simulink model "Teleoperation_Task_Space"  (R2021b)
settings: Solver=FixedStepAuto  StartTime=0.0  StopTime=20  FixedStep=Ts  RelTol=1e-3
values from neighbouring files (symbols this model uses):
  alphas_m = 75.0 * ones(1,dh.dof_task)    [setup_teleop.m]
  alphas_s = alphas_m    [setup_teleop.m]
  B_m = diag(ones(1,dh.dof_task)) * 100    [setup_teleop.m]
  B_s = diag(ones(1,dh.dof_task)) * 15    [setup_teleop.m]
  Fh_A = [1 4*wc 6*wc^2 4*wc^3 wc^4]    [setup_teleop.m]
  Fh_B = [0 0 0 0 wc^4]    [setup_teleop.m]
  gravity = [0 0 9.81]'    [setup_robot.m]
  K_g = eye(dh.dof_task) * k_g    [setup_teleop.m]
  K_m = diag(ones(1,dh.dof_task)) * 0    [setup_teleop.m]
  K_s = diag(ones(1,dh.dof_task)) * 75    [setup_teleop.m]
  KD_e = zeros(dh.dof_task); KD_e(1,1) = 10    [setup_teleop.m]
  KD_h = eye(dh.dof_task) * 50.0    [setup_teleop.m]
  KE_e = zeros(dh.dof_task); KE_e(1,1) = 100    [setup_teleop.m]
  KP_h = eye(dh.dof_task) * 350.0    [setup_teleop.m]
  lambdas_m = 4.0 * ones(1,dh.dof_task)    [setup_teleop.m]
  lambdas_s = lambdas_m    [setup_teleop.m]
  M_m = diag(ones(1,dh.dof_task)) * 1    [setup_teleop.m]
  M_s = diag(ones(1,dh.dof_task)) * 1    [setup_teleop.m]
  T_m2s = 25 / 1000 / Ts    (= 25)    [setup_teleop.m]
  T_s2m = 25 / 1000 / Ts    (= 25)    [setup_teleop.m]
  td = [            0            1                          10            18 ]    [setup_teleop.m]
  Xe = conf.init.x0    [setup_teleop.m]
  zdq_A = [1 4*wc 6*wc^2 4*wc^3 wc^4]    [setup_teleop.m]
  zdq_B = [0 0 0 0 wc^4]    [setup_teleop.m]
undefined symbols (not defined in the file or in its folder): conf_m, conf_s, dh, Fm_A, Fm_B, Fs_A, Fs_B, x0
libraries: vrlib x2, robotcorelib x1, simulink x1
(part 1 of 2)
settings Model: Creator=eros  LastModifiedBy=Sebastiano
settings SolverCC: AlgebraicLoopSolver=TrustRegion
settings DebuggingCC: SFMachineParentedDataDiag=warning

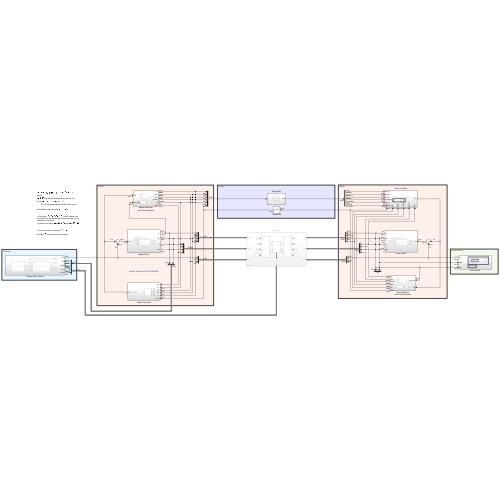
[thumbnail: Simulink's stored preview of the top-level diagram]
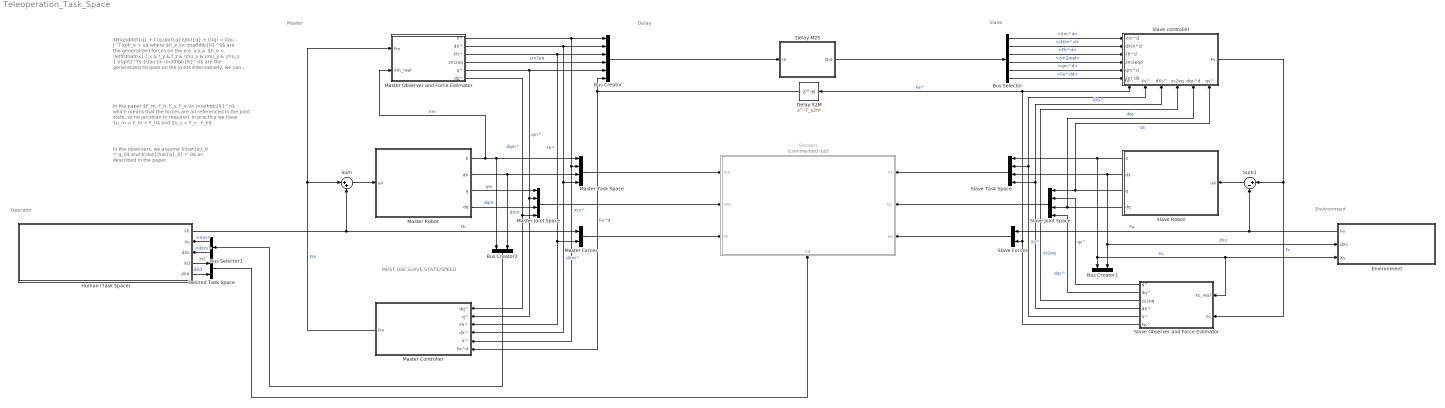
== system Teleoperation_Task_Space ==
  note: MUST USE SLAVE STATE/SPEED
  note: Operator
  note: Environment
  note: Delay
  note: Master
  note: Slave
  note: In the observers, we assume $\hat{q}_0 = q_0$ and $\dot{\hat{q}_0} = 0$ as described in the paper.
  note: In the paper $F_m, F_h, F_s, F_e \in \mathbb{R}^n$ , which means that the forces are all referenced in the joint state, so no Jacobian in required.
      | In practice we have $u_m = F_m + F_h$ and $u_s = F_s - F_e$
  note: $B(q)\ddot{q} + C(q,\dot{q})\dot{q} + G(q) = \tau - J^T(q)h_e = u$
      | where
      | $h_e \in \mathbb{R}^6$ are the generalized forces on the e.e.
      | a.k.a. $h_e = \left[\matrix{ f_x & f_y & f_z & \mu_x & \mu_y & \mu_z } \right]^T$
      | $\tau \in \mathbb{R}^n$ are the generalized torques on the joints
      |
      | Alternatively, we can write $\tau = J^T(q)\tau_e$ .
  Bus Creator : BusCreator  Inputs=6
  Bus Creator1 : BusCreator  Inputs=2
  Bus Creator2 : BusCreator  Inputs=2
  Bus Selector : BusSelector  OutputSignals=Xm^d,dXm^d,Fh^d,zm2eqd,qm^d,Fe^dd
  Bus Selector1 : BusSelector  OutputSignals=Xm,dXm
  Delay M2S : Subsystem
  Delay S2M : Delay  DelayLength=T_s2m
  Desired Task Space : BusCreator  Inputs=2
  Environment : Subsystem
      settings: PortSchema="{\"entries\":[{\"content\":{\"sides\":[{\"content\":{\"connectorIds\":[\"Out1\",\"In1\",\"In2\"]},\"type\":\"ConnectorPlacement.EquallySpacedRectSide\",\"uuid\":\"3a683f5f-8229-405f-b97f-b506986b9524\"},{\"content\":{\"connectorIds\":[],\"side\":\"RIGHT\"},\"type\":\"ConnectorPlacement.EquallySpacedRectSide\",\"uuid\":\"ee737040-7d2a-42b5-b72e-c46d7dc1a0a9\"},{\"content\":{\"connectorIds\":[],\"side\":\"TOP\"},\"type\":\"ConnectorPlacement.EquallySpacedRectSide\",\"uuid\":\"297da6e9-ed01-499d-b3c2-0f0e3cad7b3e\"}]},\"type\":\"ConnectorPlacement.EquallySpacedConnector\",\"uuid\":\"c177a36f-944e-4ac9-b62c-2e9de2d24660\"}],\"packageUris\":[\"http://schema.mathworks.com/mf0/Connector/R2020b\"],\"version\":\"1.0\"}"
  Human (Task Space) : Subsystem
      settings: PortSchema="{\"entries\":[{\"content\":{\"sides\":[{\"content\":{\"connectorIds\":[]},\"type\":\"ConnectorPlacement.EquallySpacedRectSide\",\"uuid\":\"7778f5b7-85d4-4afc-857c-056ec77f7c35\"},{\"content\":{\"connectorIds\":[\"Out1\",\"In1\",\"In2\",\"Out2\",\"Out3\"],\"side\":\"RIGHT\"},\"type\":\"ConnectorPlacement.EquallySpacedRectSide\",\"uuid\":\"4e6a4d83-f8e8-4554-84b1-926a6f2c9c17\"},{\"content\":{\"connectorIds\":[],\"side\":\"TOP\"},\"type\":\"ConnectorPlacement.EquallySpacedRectSide\",\"uuid\":\"7c53f63a-15b9-4620-895a-15c4690edfa5\"}]},\"type\":\"ConnectorPlacement.EquallySpacedConnector\",\"uuid\":\"f47fbd83-fa7b-4372-bf8b-e8c7b2e83c33\"}],\"packageUris\":[\"http://schema.mathworks.com/mf0/Connector/R2020b\"],\"version\":\"1.0\"}"
  Master Controller : Subsystem
  Master Forces : BusCreator  Inputs=2
  Master Joint Space : BusCreator  Inputs=4
  Master Observer and Force Estimator : Subsystem
  Master Robot : Subsystem
  Master Task Space : BusCreator  Inputs=4
  Sensors : Subsystem  Commented=on
      settings: PortSchema="{\"entries\":[{\"content\":{\"sides\":[{\"content\":{\"connectorIds\":[\"In1\",\"In2\",\"In3\"]},\"type\":\"ConnectorPlacement.EquallySpacedRectSide\",\"uuid\":\"54c087a6-e628-45a0-8beb-ec377517c1fd\"},{\"content\":{\"connectorIds\":[\"In5\",\"In6\",\"In7\"],\"side\":\"RIGHT\"},\"type\":\"ConnectorPlacement.EquallySpacedRectSide\",\"uuid\":\"42defee6-bb8f-41f0-bcac-2060d15fab8b\"},{\"content\":{\"connectorIds\":[],\"side\":\"TOP\"},\"type\":\"ConnectorPlacement.EquallySpacedRectSide\",\"uuid\":\"25403ab0-b6a1-4ec4-8138-b166c3bde76b\"},{\"content\":{\"connectorIds\":[\"In4\"],\"side\":\"BOTTOM\"},\"type\":\"ConnectorPlacement.EquallySpacedRectSide\",\"uuid\":\"d9d00fac-eb94-4801-95c9-2f27ca054ba8\"}]},\"type\":\"ConnectorPlacement.EquallySpacedConnector\",\"uuid\":\"2fd4c0cb-09a7-477d-a6ac-6df7d0139477\"}],\"packageUris\":[\"http://schema.mathworks.com/mf0/Connector/R2020b\"],\"version\":\"1.0\"}"
  Slave Forces : BusCreator  Inputs=2
  Slave Joint Space : BusCreator  Inputs=4
  Slave Observer and Force Estimator : Subsystem
  Slave Robot : Subsystem
  Slave Task Space : BusCreator  Inputs=4
  Slave controller : Subsystem
      settings: PortSchema="{\"entries\":[{\"content\":{\"sides\":[{\"content\":{\"connectorIds\":[\"In1\",\"In2\",\"In3\",\"In4\",\"In5\",\"In6\"]},\"type\":\"ConnectorPlacement.EquallySpacedRectSide\",\"uuid\":\"b1f66af2-ed99-40b6-8cf8-b97c23f93a67\"},{\"content\":{\"connectorIds\":[\"Out1\"],\"side\":\"RIGHT\"},\"type\":\"ConnectorPlacement.EquallySpacedRectSide\",\"uuid\":\"bd8dc41a-d4bd-4421-a4e6-8b9f2d2ea86c\"},{\"content\":{\"connectorIds\":[],\"side\":\"TOP\"},\"type\":\"ConnectorPlacement.EquallySpacedRectSide\",\"uuid\":\"bc806d3a-77b0-4d29-b087-7d48d5aabf51\"},{\"content\":{\"connectorIds\":[\"In7\",\"In8\",\"In9\",\"In10\",\"In11\",\"In12\"],\"side\":\"BOTTOM\"},\"type\":\"ConnectorPlacement.EquallySpacedRectSide\",\"uuid\":\"ca1d5307-1d0f-4028-b8dc-88a57f95ff6b\"}]},\"type\":\"ConnectorPlacement.EquallySpacedConnector\",\"uuid\":\"a48c829b-f218-4f75-a112-dfe3646c5e86\"}],\"packageUris\":[\"http://schema.mathworks.com/mf0/Connector/R2020b\"],\"version\":\"1.0\"}"
  Sum : Sum  Inputs=|++
  Sum1 : Sum  Inputs=|+-
  wires:
  Slave Observer and Force Estimator/1(q^) -> Slave Joint Space/2  "qs^"
  Slave Observer and Force Estimator/3(zs2eq) -> Slave controller/10(zs2eq)  "zs2eq"
  Master Observer and Force Estimator/1(X^) -> Master Task Space/2, Master Controller/5(X^), Bus Creator/1  "Xm^"
  Slave Observer and Force Estimator/6(Fe^) -> Delay S2M/1, Slave controller/7(Fe^), Slave Forces/2  "Fe^"
  Master Observer and Force Estimator/3(Fh^) -> Bus Creator/3, Master Controller/3(Fh^), Master Forces/2  "Fh^"
  Slave Observer and Force Estimator/2(dq^) -> Slave Joint Space/4  "dqs^"
  Master Observer and Force Estimator/2(dX^) -> Bus Creator/2, Master Task Space/4, Master Controller/4(dX^)  "dXm^"
  Master Controller/1(Fm) -> Master Observer and Force Estimator/1(Fm), Sum/1  "Fm"
  Slave controller/1(Fs) -> Slave Observer and Force Estimator/2(Fs), Sum1/1  "Fs"
  Master Observer and Force Estimator/4(zm2eq) -> Bus Creator/4  "zm2eq"
  Bus Selector/6 -> Slave controller/6(Fe^dd)  "<Fe^dd>"
  Bus Selector/2 -> Slave controller/2(dXm^d)  "<dXm^d>"
  Bus Selector/1 -> Slave controller/1(Xm^d)  "<Xm^d>"
  Bus Selector/3 -> Slave controller/3(Fh^d)  "<Fh^d>"
  Bus Selector/4 -> Slave controller/4(zm2eqd)  "<zm2eqd>"
  Delay S2M/1 -> Bus Creator/6, Master Controller/6(Fe^d)  "Fe^d"
  Slave Robot/3(q) -> Slave Joint Space/1, Slave controller/12(qs^)  "qs"
  Slave Robot/4(dq) -> Slave Joint Space/3, Slave controller/11(dqs^d)  "dqs"
  Master Robot/1(X) -> Bus Creator2/1, Master Task Space/1, Master Observer and Force Estimator/2(Xm_real)  "Xm"
  Human (Task Space)/1(Fh) -> Sum/2, Master Forces/1  "Fh"
  Sum/1 -> Master Robot/1(uA)
  Master Robot/3(q) -> Master Joint Space/1  "qm"
  Master Observer and Force Estimator/5(q^) -> Bus Creator/5, Master Controller/2(q^), Master Joint Space/2  "qm^"
  Master Observer and Force Estimator/6(dq^) -> Master Controller/1(dq^), Master Joint Space/4  "dqm^"
  Master Robot/4(dq) -> Master Joint Space/3  "dqm"
  Master Robot/2(dX) -> Master Task Space/3, Bus Creator2/2  "dXm"
  Sum1/1 -> Slave Robot/1(uA)
  Slave Robot/1(X) -> Slave Observer and Force Estimator/1(Xs_real), Environment/2(Xs), Bus Creator1/1, Slave Task Space/1  "Xs"
  Slave Robot/2(dX) -> Slave Task Space/3, Environment/1(dXs), Bus Creator1/2  "dXs"
  Slave Observer and Force Estimator/5(X^) -> Slave controller/8(Xs^), Slave Task Space/2  "Xs^"
  Slave Observer and Force Estimator/4(dX^) -> Slave Task Space/4, Slave controller/9(dXs^)  "dXs^"
  Bus Selector/5 -> Slave controller/5(qm^d)  "<qm^d>"
  Environment/1(Fe) -> Sum1/2, Slave Forces/1  "Fe"
  Human (Task Space)/2(Xd) -> Desired Task Space/1  "Xd"
  Human (Task Space)/3(dXd) -> Desired Task Space/2  "dXd"
  Master Task Space/1 -> Sensors/1(Xm)
  Slave Task Space/1 -> Sensors/5(Xs)
  Master Joint Space/1 -> Sensors/2(Qm)
  Slave Joint Space/1 -> Sensors/6(Qs)
  Master Forces/1 -> Sensors/3(Fh)
  Slave Forces/1 -> Sensors/7(Fe)
  Desired Task Space/1 -> Sensors/4(Xd)
  Bus Selector1/2 -> Human (Task Space)/2(dXs)  "<dXm>"
  Bus Selector1/1 -> Human (Task Space)/1(Xs)  "<Xm>"
  Bus Creator2/1 -> Bus Selector1/1
  Bus Creator/1 -> Delay M2S/1(In)
  Delay M2S/1(Out) -> Bus Selector/1

== system Teleoperation_Task_Space/Delay M2S ==
  note: Initial conditions of the delays are set to be the initial condition of the slave robot.
      | When the first signal from the master is received, the slave follows it immediately.
  In : Inport
  Bus Creator3 : BusCreator  Inputs=6
  Bus Selector2 : BusSelector  OutputSignals=Xm^,dXm^,Fh^,zm2eq,qm^,Fe^d
  Delay M2S : Delay  DelayLength=T_m2s  InitialCondition=repmat(conf_s.init.x0, [1,1,T_m2s])
  Delay M2S1 : Delay  DelayLength=T_m2s
  Delay M2S2 : Delay  DelayLength=T_m2s  InitialCondition=repmat(conf_s.init.q0, [1,T_m2s])
  Delay M2S3 : Delay  DelayLength=T_m2s
  Delay M2S4 : Delay  DelayLength=T_m2s
  Delay M2S5 : Delay  DelayLength=T_m2s  InitialCondition=repmat(conf_s.init.dx0, [1,1,T_m2s])
  Out : Outport
  wires:
  Delay M2S4/1 -> Bus Creator3/3  "Fh^d"
  Bus Selector2/4 -> Delay M2S3/1  "<zm2eq>"
  Delay M2S2/1 -> Bus Creator3/5  "qm^d"
  Delay M2S3/1 -> Bus Creator3/4  "zm2eqd"
  Bus Selector2/1 -> Delay M2S/1  "<Xm^>"
  Bus Selector2/5 -> Delay M2S2/1  "<qm^>"
  Delay M2S5/1 -> Bus Creator3/2  "dXm^d"
  Bus Selector2/6 -> Delay M2S1/1  "<Fe^d>"
  Delay M2S1/1 -> Bus Creator3/6  "Fe^dd"
  Bus Selector2/2 -> Delay M2S5/1  "<dXm^>"
  Bus Selector2/3 -> Delay M2S4/1  "<Fh^>"
  Delay M2S/1 -> Bus Creator3/1  "Xm^d"
  In/1 -> Bus Selector2/1
  Bus Creator3/1 -> Out/1

== system Teleoperation_Task_Space/Environment ==
  note: No Environment
  note: Spring Environment
  note: Spring-Damper Environment
  dXs : Inport
  Xs : Inport  Port=2
  Constant1 : Constant  Value=zeros(1,dh.dof_task)
  Constant2 : Constant  Value=zeros(1,dh.dof_task)
  Constant4 : Constant  Value=Xe
  Manual Switch : ManualSwitch
  Manual Switch1 : ManualSwitch
  Multiply : Gain  Gain=KE_e  Multiplication=Matrix(K*u)
  Multiply1 : Gain  Gain=KD_e  Multiplication=Matrix(K*u)
  Product : Product
  Subsystem : Subsystem
  Sum : Sum  Inputs=|++
  Fe : Outport
  wires:
  Product/1 -> Manual Switch/1
  Constant1/1 -> Manual Switch1/2
  Manual Switch/1 -> Fe/1
  Multiply/1 -> Sum/1
  Manual Switch1/1 -> Sum/2
  Multiply1/1 -> Manual Switch1/1
  dXs/1 -> Multiply1/1
  Constant2/1 -> Manual Switch/2
  Constant4/1 -> Subsystem/2(EnvironmentPose)
  Xs/1 -> Subsystem/1(SlavePose)
  Subsystem/1(IsTouching) -> Product/1
  Sum/1 -> Product/2
  Subsystem/2(Displacement) -> Multiply/1

== system Teleoperation_Task_Space/Human (Task Space) ==
  Xs : Inport
  dXs : Inport  Port=2
  Motion Tracking control : Subsystem
      settings: PortSchema="{\"entries\":[{\"content\":{\"sides\":[{\"content\":{\"connectorIds\":[\"In1\",\"In2\",\"In3\"]},\"type\":\"ConnectorPlacement.EquallySpacedRectSide\",\"uuid\":\"52575601-e286-4809-a30d-cedf982d9693\"},{\"content\":{\"connectorIds\":[\"Out1\",\"In4\",\"In5\"],\"side\":\"RIGHT\"},\"type\":\"ConnectorPlacement.EquallySpacedRectSide\",\"uuid\":\"ad2168cb-d0b7-4f4a-9914-0c84d01558f7\"},{\"content\":{\"connectorIds\":[],\"side\":\"TOP\"},\"type\":\"ConnectorPlacement.EquallySpacedRectSide\",\"uuid\":\"311024f8-e557-4a51-82a2-8dec63492c2b\"}]},\"type\":\"ConnectorPlacement.EquallySpacedConnector\",\"uuid\":\"f15c02cd-b134-4f17-b903-786a9234fd9d\"}],\"packageUris\":[\"http://schema.mathworks.com/mf0/Connector/R2020b\"],\"version\":\"1.0\"}"
  Task Space trajectory : Subsystem
  Fh : Outport
  Xd : Outport  Port=2
  dXd : Outport  Port=3
  wires:
  Task Space trajectory/2(dXd) -> dXd/1, Motion Tracking control/2(dXd)
  dXs/1 -> Motion Tracking control/4(dXs)
  Motion Tracking control/1(uA) -> Fh/1
  Xs/1 -> Motion Tracking control/5(Xs)
  Task Space trajectory/3(Xd) -> Xd/1, Motion Tracking control/3(Xd)
  Task Space trajectory/1(ddXd) -> Motion Tracking control/1(ddXd)

== system Teleoperation_Task_Space/Master Controller ==
  note: Here we provide q^ and dq^ just to avoid calculating them
  dq^ : Inport
  q^ : Inport  Port=2
  Fh^ : Inport  Port=3
  dX^ : Inport  Port=4
  X^ : Inport  Port=5
  Fe^d : Inport  Port=6
  Master Command Filter : Subsystem  Commented=through  TreatAsAtomicUnit=on
  Master Controller : MATLAB Function  TreatAsAtomicUnit=on
  Fm : Outport
  wires:
  Fh^/1 -> Master Controller/5(Fh)
  Fe^d/1 -> Master Controller/6(Fe_d)
  Master Controller/1(Fm) -> Master Command Filter/1(In1)
  X^/1 -> Master Controller/3(Xm)
  dX^/1 -> Master Controller/4(dXm)
  dq^/1 -> Master Controller/2(dqm)
  q^/1 -> Master Controller/1(qm)
  Master Command Filter/1(Out1) -> Fm/1

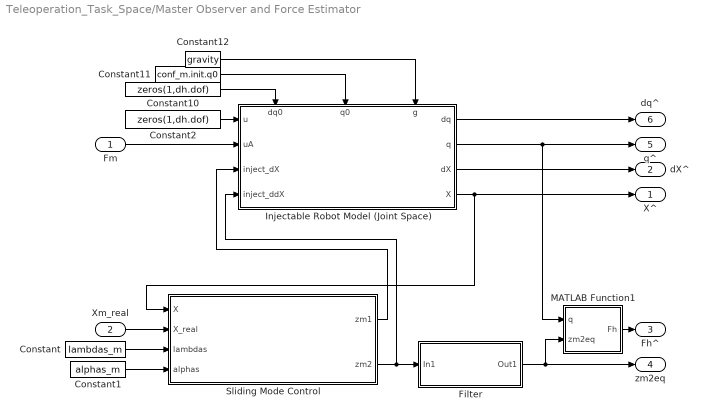
== system Teleoperation_Task_Space/Master Observer and Force Estimator ==
  Fm : Inport
  Xm_real : Inport  Port=2
  Constant : Constant  Value=lambdas_m
  Constant1 : Constant  Value=alphas_m
  Constant10 : Constant  Value=zeros(1,dh.dof)
  Constant11 : Constant  Value=conf_m.init.q0
  Constant12 : Constant  Value=gravity
  Constant2 : Constant  Value=zeros(1,dh.dof)
  Filter : Subsystem  TreatAsAtomicUnit=on
  Injectable Robot Model (Joint Space) : Subsystem
      settings: PortSchema="{\"entries\":[{\"content\":{\"sides\":[{\"content\":{\"connectorIds\":[\"In1\",\"In2\",\"In3\",\"In4\"]},\"type\":\"ConnectorPlacement.EquallySpacedRectSide\",\"uuid\":\"a8701c64-329e-4144-b882-ecf5d621aff2\"},{\"content\":{\"connectorIds\":[\"Out1\",\"Out2\",\"Out3\",\"Out4\"],\"side\":\"RIGHT\"},\"type\":\"ConnectorPlacement.EquallySpacedRectSide\",\"uuid\":\"4e168703-1cb9-438c-bc6b-9b2d7fbb809e\"},{\"content\":{\"connectorIds\":[\"In5\",\"In6\",\"In7\"],\"side\":\"TOP\"},\"type\":\"ConnectorPlacement.EquallySpacedRectSide\",\"uuid\":\"8fbcb29e-7fab-4224-b4ad-ee01c13d675a\"}]},\"type\":\"ConnectorPlacement.EquallySpacedConnector\",\"uuid\":\"fa721fab-1ce6-4fdf-95fa-8ada3ed2d65c\"}],\"packageUris\":[\"http://schema.mathworks.com/mf0/Connector/R2020b\"],\"version\":\"1.0\"}"
  MATLAB Function1 : MATLAB Function  TreatAsAtomicUnit=on
  Sliding Mode Control : Subsystem
  X^ : Outport
  dX^ : Outport  Port=2
  Fh^ : Outport  Port=3
  zm2eq : Outport  Port=4
  q^ : Outport  Port=5
  dq^ : Outport  Port=6
  wires:
  Filter/1(Out1) -> MATLAB Function1/2(zm2eq), zm2eq/1
  Sliding Mode Control/1(zm1) -> Injectable Robot Model (Joint Space)/3(inject_dX)
  Sliding Mode Control/2(zm2) -> Filter/1(In1), Injectable Robot Model (Joint Space)/4(inject_ddX)
  Constant1/1 -> Sliding Mode Control/4(alphas)
  Constant/1 -> Sliding Mode Control/3(lambdas)
  Xm_real/1 -> Sliding Mode Control/2(X_real)
  Injectable Robot Model (Joint Space)/4(X) -> X^/1, Sliding Mode Control/1(X)
  Injectable Robot Model (Joint Space)/3(dX) -> dX^/1
  Constant11/1 -> Injectable Robot Model (Joint Space)/6(q0)
  Constant10/1 -> Injectable Robot Model (Joint Space)/5(dq0)
  Injectable Robot Model (Joint Space)/1(dq) -> dq^/1
  Constant12/1 -> Injectable Robot Model (Joint Space)/7(g)
  Injectable Robot Model (Joint Space)/2(q) -> MATLAB Function1/1(q), q^/1
  MATLAB Function1/1(Fh) -> Fh^/1
  Constant2/1 -> Injectable Robot Model (Joint Space)/1(u)
  Fm/1 -> Injectable Robot Model (Joint Space)/2(uA)

== system Teleoperation_Task_Space/Master Robot ==
  uA : Inport
  Constant1 : Constant  Value=zeros(1,dh.dof)
  Constant10 : Constant  Value=conf_m.init.dq0
  Constant11 : Constant  Value=conf_m.init.q0
  Constant12 : Constant  Value=gravity
  Constant2 : Constant  Value=zeros(1,dh.dof_task)
  Injectable Robot Model (Joint Space) : Subsystem
      settings: PortSchema="{\"entries\":[{\"content\":{\"sides\":[{\"content\":{\"connectorIds\":[\"In1\",\"In2\",\"In3\",\"In4\"]},\"type\":\"ConnectorPlacement.EquallySpacedRectSide\",\"uuid\":\"a8701c64-329e-4144-b882-ecf5d621aff2\"},{\"content\":{\"connectorIds\":[\"Out1\",\"Out2\",\"Out3\",\"Out4\"],\"side\":\"RIGHT\"},\"type\":\"ConnectorPlacement.EquallySpacedRectSide\",\"uuid\":\"4e168703-1cb9-438c-bc6b-9b2d7fbb809e\"},{\"content\":{\"connectorIds\":[\"In5\",\"In6\",\"In7\"],\"side\":\"TOP\"},\"type\":\"ConnectorPlacement.EquallySpacedRectSide\",\"uuid\":\"8fbcb29e-7fab-4224-b4ad-ee01c13d675a\"}]},\"type\":\"ConnectorPlacement.EquallySpacedConnector\",\"uuid\":\"fa721fab-1ce6-4fdf-95fa-8ada3ed2d65c\"}],\"packageUris\":[\"http://schema.mathworks.com/mf0/Connector/R2020b\"],\"version\":\"1.0\"}"
  X : Outport
  dX : Outport  Port=2
  q : Outport  Port=3
  dq : Outport  Port=4
  wires:
  Constant10/1 -> Injectable Robot Model (Joint Space)/5(dq0)
  Constant2/1 -> Injectable Robot Model (Joint Space)/4(inject_ddX), Injectable Robot Model (Joint Space)/3(inject_dX)
  Constant11/1 -> Injectable Robot Model (Joint Space)/6(q0)
  Injectable Robot Model (Joint Space)/2(q) -> q/1
  Injectable Robot Model (Joint Space)/3(dX) -> dX/1
  Constant12/1 -> Injectable Robot Model (Joint Space)/7(g)
  Injectable Robot Model (Joint Space)/4(X) -> X/1
  Injectable Robot Model (Joint Space)/1(dq) -> dq/1
  uA/1 -> Injectable Robot Model (Joint Space)/2(uA)
  Constant1/1 -> Injectable Robot Model (Joint Space)/1(u)

== system Teleoperation_Task_Space/Sensors ==
  Xm : Inport
  Qm : Inport  Port=2
  Fh : Inport  Port=3
  Xd : Inport  Port=4
  Xs : Inport  Port=5
  Qs : Inport  Port=6
  Fe : Inport  Port=7
  Compare Sensors : Subsystem
      settings: PortSchema="{\"entries\":[{\"content\":{\"sides\":[{\"content\":{\"connectorIds\":[\"In1\",\"In2\"]},\"type\":\"ConnectorPlacement.EquallySpacedRectSide\",\"uuid\":\"eee4eb85-6cb8-4462-85fc-1aafb3c3937f\"},{\"content\":{\"connectorIds\":[\"In4\",\"In5\"],\"side\":\"RIGHT\"},\"type\":\"ConnectorPlacement.EquallySpacedRectSide\",\"uuid\":\"5ab37ec6-6ee1-47e9-aff6-41baaee9b59b\"},{\"content\":{\"connectorIds\":[],\"side\":\"TOP\"},\"type\":\"ConnectorPlacement.EquallySpacedRectSide\",\"uuid\":\"6f11ee79-2d90-4b50-8360-b99d360f33b3\"},{\"content\":{\"connectorIds\":[\"In3\"],\"side\":\"BOTTOM\"},\"type\":\"ConnectorPlacement.EquallySpacedRectSide\",\"uuid\":\"fafd6e14-ac6f-4eee-8610-fc1b1c686699\"}]},\"type\":\"ConnectorPlacement.EquallySpacedConnector\",\"uuid\":\"5676dc65-12f4-4a54-a0ce-a07c6c462ad2\"}],\"packageUris\":[\"http://schema.mathworks.com/mf0/Connector/R2020b\"],\"version\":\"1.0\"}"
  Master Desired Pose : Subsystem
  Master Sensors : Subsystem
  Slave Desired Pose : Subsystem
  Slave Sensors : Subsystem
  wires:
  Xd/1 -> Compare Sensors/3(Xd)
  Slave Sensors/2(dXs) -> Compare Sensors/5(dXs)
  Master Sensors/2(dXm) -> Compare Sensors/2(dXm)
  Fh/1 -> Master Sensors/3(F)
  Fe/1 -> Slave Sensors/3(F)
  Qs/1 -> Slave Sensors/2(Q)
  Xm/1 -> Master Sensors/1(X)
  Master Sensors/1(Xm) -> Compare Sensors/1(Xm)
  Slave Sensors/1(Xs) -> Compare Sensors/4(Xs)
  Qm/1 -> Master Sensors/2(Q)
  Xs/1 -> Slave Sensors/1(X)
  Slave Desired Pose/1(Xd) -> Slave Sensors/4(Xd)
  Master Desired Pose/1(Xd) -> Master Sensors/4(Xd)

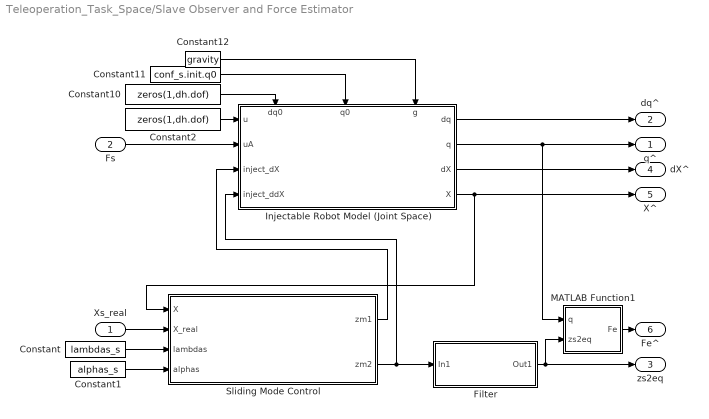
== system Teleoperation_Task_Space/Slave Observer and Force Estimator ==
  Xs_real : Inport
  Fs : Inport  Port=2
  Constant : Constant  Value=lambdas_s
  Constant1 : Constant  Value=alphas_s
  Constant10 : Constant  Value=zeros(1,dh.dof)
  Constant11 : Constant  Value=conf_s.init.q0
  Constant12 : Constant  Value=gravity
  Constant2 : Constant  Value=zeros(1,dh.dof)
  Filter : Subsystem  TreatAsAtomicUnit=on
  Injectable Robot Model (Joint Space) : Subsystem
      settings: PortSchema="{\"entries\":[{\"content\":{\"sides\":[{\"content\":{\"connectorIds\":[\"In1\",\"In2\",\"In3\",\"In4\"]},\"type\":\"ConnectorPlacement.EquallySpacedRectSide\",\"uuid\":\"a8701c64-329e-4144-b882-ecf5d621aff2\"},{\"content\":{\"connectorIds\":[\"Out1\",\"Out2\",\"Out3\",\"Out4\"],\"side\":\"RIGHT\"},\"type\":\"ConnectorPlacement.EquallySpacedRectSide\",\"uuid\":\"4e168703-1cb9-438c-bc6b-9b2d7fbb809e\"},{\"content\":{\"connectorIds\":[\"In5\",\"In6\",\"In7\"],\"side\":\"TOP\"},\"type\":\"ConnectorPlacement.EquallySpacedRectSide\",\"uuid\":\"8fbcb29e-7fab-4224-b4ad-ee01c13d675a\"}]},\"type\":\"ConnectorPlacement.EquallySpacedConnector\",\"uuid\":\"fa721fab-1ce6-4fdf-95fa-8ada3ed2d65c\"}],\"packageUris\":[\"http://schema.mathworks.com/mf0/Connector/R2020b\"],\"version\":\"1.0\"}"
  MATLAB Function1 : MATLAB Function  TreatAsAtomicUnit=on
  Sliding Mode Control : Subsystem
  q^ : Outport
  dq^ : Outport  Port=2
  zs2eq : Outport  Port=3
  dX^ : Outport  Port=4
  X^ : Outport  Port=5
  Fe^ : Outport  Port=6
  wires:
  Filter/1(Out1) -> MATLAB Function1/2(zs2eq), zs2eq/1
  Sliding Mode Control/1(zm1) -> Injectable Robot Model (Joint Space)/3(inject_dX)
  Sliding Mode Control/2(zm2) -> Filter/1(In1), Injectable Robot Model (Joint Space)/4(inject_ddX)
  Constant1/1 -> Sliding Mode Control/4(alphas)
  Constant/1 -> Sliding Mode Control/3(lambdas)
  Xs_real/1 -> Sliding Mode Control/2(X_real)
  Injectable Robot Model (Joint Space)/4(X) -> Sliding Mode Control/1(X), X^/1
  Injectable Robot Model (Joint Space)/3(dX) -> dX^/1
  Constant11/1 -> Injectable Robot Model (Joint Space)/6(q0)
  Constant10/1 -> Injectable Robot Model (Joint Space)/5(dq0)
  Injectable Robot Model (Joint Space)/1(dq) -> dq^/1
  Constant12/1 -> Injectable Robot Model (Joint Space)/7(g)
  Injectable Robot Model (Joint Space)/2(q) -> MATLAB Function1/1(q), q^/1
  MATLAB Function1/1(Fe) -> Fe^/1
  Constant2/1 -> Injectable Robot Model (Joint Space)/1(u)
  Fs/1 -> Injectable Robot Model (Joint Space)/2(uA)

== system Teleoperation_Task_Space/Slave Robot ==
  uA : Inport
  Constant1 : Constant  Value=zeros(1,dh.dof)
  Constant10 : Constant  Value=conf_s.init.dq0
  Constant11 : Constant  Value=conf_s.init.q0
  Constant12 : Constant  Value=gravity
  Constant2 : Constant  Value=zeros(1,dh.dof_task)
  Injectable Robot Model (Joint Space) : Subsystem
      settings: PortSchema="{\"entries\":[{\"content\":{\"sides\":[{\"content\":{\"connectorIds\":[\"In1\",\"In2\",\"In3\",\"In4\"]},\"type\":\"ConnectorPlacement.EquallySpacedRectSide\",\"uuid\":\"a8701c64-329e-4144-b882-ecf5d621aff2\"},{\"content\":{\"connectorIds\":[\"Out1\",\"Out2\",\"Out3\",\"Out4\"],\"side\":\"RIGHT\"},\"type\":\"ConnectorPlacement.EquallySpacedRectSide\",\"uuid\":\"4e168703-1cb9-438c-bc6b-9b2d7fbb809e\"},{\"content\":{\"connectorIds\":[\"In5\",\"In6\",\"In7\"],\"side\":\"TOP\"},\"type\":\"ConnectorPlacement.EquallySpacedRectSide\",\"uuid\":\"8fbcb29e-7fab-4224-b4ad-ee01c13d675a\"}]},\"type\":\"ConnectorPlacement.EquallySpacedConnector\",\"uuid\":\"fa721fab-1ce6-4fdf-95fa-8ada3ed2d65c\"}],\"packageUris\":[\"http://schema.mathworks.com/mf0/Connector/R2020b\"],\"version\":\"1.0\"}"
  X : Outport
  dX : Outport  Port=2
  q : Outport  Port=3
  dq : Outport  Port=4
  wires:
  Constant10/1 -> Injectable Robot Model (Joint Space)/5(dq0)
  Constant2/1 -> Injectable Robot Model (Joint Space)/4(inject_ddX), Injectable Robot Model (Joint Space)/3(inject_dX)
  Constant11/1 -> Injectable Robot Model (Joint Space)/6(q0)
  Injectable Robot Model (Joint Space)/2(q) -> q/1
  Injectable Robot Model (Joint Space)/3(dX) -> dX/1
  Constant12/1 -> Injectable Robot Model (Joint Space)/7(g)
  Injectable Robot Model (Joint Space)/4(X) -> X/1
  Injectable Robot Model (Joint Space)/1(dq) -> dq/1
  uA/1 -> Injectable Robot Model (Joint Space)/2(uA)
  Constant1/1 -> Injectable Robot Model (Joint Space)/1(u)

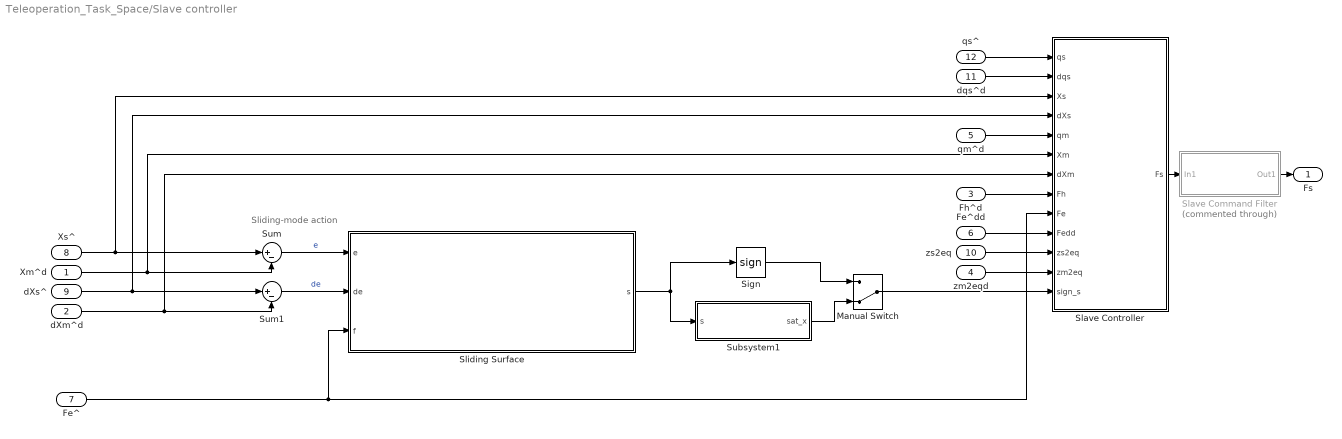
== system Teleoperation_Task_Space/Slave controller ==
  note: Sliding-mode action
  Xm^d : Inport
  dXm^d : Inport  Port=2
  Fh^d : Inport  Port=3
  zm2eqd : Inport  Port=4
  qm^d : Inport  Port=5
  Fe^dd : Inport  Port=6
  Fe^ : Inport  Port=7
  Xs^ : Inport  Port=8
  dXs^ : Inport  Port=9
  zs2eq : Inport  Port=10
  dqs^d : Inport  Port=11
  qs^ : Inport  Port=12
  Manual Switch : ManualSwitch  CurrentSetting=0
  Sign : Signum
  Slave Command Filter : Subsystem  Commented=through  TreatAsAtomicUnit=on
  Slave Controller : MATLAB Function  TreatAsAtomicUnit=on
  Sliding Surface : Subsystem
  Subsystem1 : Subsystem
  Sum : Sum  Inputs=|+-
  Sum1 : Sum  Inputs=|+-
  Fs : Outport
  wires:
  zs2eq/1 -> Slave Controller/11(zs2eq)
  Fh^d/1 -> Slave Controller/8(Fh)
  Slave Controller/1(Fs) -> Slave Command Filter/1(In1)
  zm2eqd/1 -> Slave Controller/12(zm2eq)
  Fe^dd/1 -> Slave Controller/10(Fedd)
  Xs^/1 -> Slave Controller/3(Xs), Sum/1
  Xm^d/1 -> Sum/2, Slave Controller/6(Xm)
  dXs^/1 -> Slave Controller/4(dXs), Sum1/1
  dXm^d/1 -> Sum1/2, Slave Controller/7(dXm)
  Fe^/1 -> Sliding Surface/3(f), Slave Controller/9(Fe)
  Sign/1 -> Manual Switch/1
  Sum/1 -> Sliding Surface/1(e)  "e"
  Sum1/1 -> Sliding Surface/2(de)  "de"
  Sliding Surface/1(s) -> Subsystem1/1(s), Sign/1
  Subsystem1/1(sat_x) -> Manual Switch/2
  Manual Switch/1 -> Slave Controller/13(sign_s)
  qs^/1 -> Slave Controller/1(qs)
  dqs^d/1 -> Slave Controller/2(dqs)
  qm^d/1 -> Slave Controller/5(qm)
  Slave Command Filter/1(Out1) -> Fs/1

== system Teleoperation_Task_Space/Environment/Subsystem ==
  SlavePose : Inport
  EnvironmentPose : Inport  Port=2
  Constant2 : Constant  Value=zeros(1,dh.dof_task)
  Min : MinMax  Function=max  Inputs=2
  Sign : Signum
  Sum2 : Sum  Inputs=|-+
  IsTouching : Outport
  Displacement : Outport  Port=2
  wires:
  Constant2/1 -> Min/2
  Sum2/1 -> Displacement/1, Min/1
  SlavePose/1 -> Sum2/2
  Min/1 -> Sign/1
  EnvironmentPose/1 -> Sum2/1
  Sign/1 -> IsTouching/1

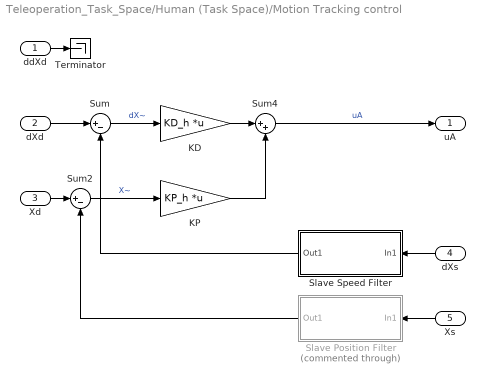
== system Teleoperation_Task_Space/Human (Task Space)/Motion Tracking control ==
  ddXd : Inport
  dXd : Inport  Port=2
  Xd : Inport  Port=3
  dXs : Inport  Port=4
  Xs : Inport  Port=5
  KD : Gain  Gain=KD_h  Multiplication=Matrix(K*u)
  KP : Gain  Gain=KP_h  Multiplication=Matrix(K*u)
  Slave Position Filter : Subsystem  Commented=through  TreatAsAtomicUnit=on
  Slave Speed Filter : Subsystem  TreatAsAtomicUnit=on
  Sum : Sum  Inputs=|+-
  Sum2 : Sum  Inputs=|+-
  Sum4 : Sum  Inputs=|++
  Terminator : Terminator
  uA : Outport
  wires:
  Xd/1 -> Sum2/1
  KP/1 -> Sum4/2
  Sum4/1 -> uA/1  "uA"
  Slave Speed Filter/1(Out1) -> Sum/2
  Xs/1 -> Slave Position Filter/1(In1)
  Sum2/1 -> KP/1  "X~"
  KD/1 -> Sum4/1
  Sum/1 -> KD/1  "dX~"
  dXd/1 -> Sum/1
  ddXd/1 -> Terminator/1
  dXs/1 -> Slave Speed Filter/1(In1)
  Slave Position Filter/1(Out1) -> Sum2/2

== system Teleoperation_Task_Space/Human (Task Space)/Task Space trajectory ==
  Polynomial Trajectory : robotcorelib/Polynomial Trajectory  WaypointSource=Internal  Waypoints=Xd  TimePoints=td  TimeInterval=[ 1, 4 ]  Method=Cubic Polynomial  ParameterSource=Internal  VelocityBoundaryCondition=zeros(dh.dof_task, length(td))  AccelerationBoundaryCondition=zeros( 2, 5 )  SimulateUsing=Code generation
  Ramp : simulink/Sources/Ramp  slope=1  start=0  InitialOutput=0
  ddXd : Outport
  dXd : Outport  Port=2
  Xd : Outport  Port=3
  wires:
  Polynomial Trajectory/1 -> Xd/1
  Polynomial Trajectory/2 -> dXd/1
  Ramp/1 -> Polynomial Trajectory/1
  Polynomial Trajectory/3 -> ddXd/1

== system Teleoperation_Task_Space/Master Controller/Master Command Filter ==
  In1 : Inport  Partition=on  PartitionDimension=1  PartitionWidth=1  PartitionOffset=0
  Filter : TransferFcn  Numerator=Fm_B  Denominator=Fm_A
  For Each : ForEach  DisableCoverage=on
  Out1 : Outport  ConcatenationDimension=1
  wires:
  In1/1 -> Filter/1
  Filter/1 -> Out1/1

== system Teleoperation_Task_Space/Master Observer and Force Estimator/Filter ==
  In1 : Inport  Partition=on  PartitionDimension=1  PartitionWidth=1  PartitionOffset=0
  Filter : TransferFcn  Numerator=zdq_B  Denominator=zdq_A
  For Each : ForEach  DisableCoverage=on
  Out1 : Outport  ConcatenationDimension=1
  wires:
  In1/1 -> Filter/1
  Filter/1 -> Out1/1

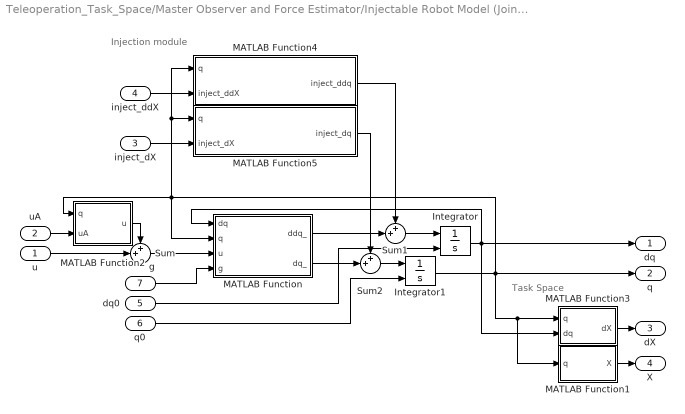
== system Teleoperation_Task_Space/Master Observer and Force Estimator/Injectable Robot Model (Joint Space) ==
  note: Injection module
  note: Task Space
  u : Inport
  uA : Inport  Port=2
  inject_dX : Inport  Port=3
  inject_ddX : Inport  Port=4
  dq0 : Inport  Port=5
  q0 : Inport  Port=6
  g : Inport  Port=7
  Integrator : Integrator  InitialConditionSource=external  InitialCondition=x0
  Integrator1 : Integrator  InitialConditionSource=external  InitialCondition=x0
  MATLAB Function : MATLAB Function  TreatAsAtomicUnit=on
  MATLAB Function1 : MATLAB Function  TreatAsAtomicUnit=on
  MATLAB Function2 : MATLAB Function  TreatAsAtomicUnit=on
  MATLAB Function3 : MATLAB Function  TreatAsAtomicUnit=on
  MATLAB Function4 : MATLAB Function  TreatAsAtomicUnit=on
  MATLAB Function5 : MATLAB Function  TreatAsAtomicUnit=on
  Sum : Sum  Inputs=++|
  Sum1 : Sum  Inputs=++|
  Sum2 : Sum  Inputs=++|
  dq : Outport
  q : Outport  Port=2
  dX : Outport  Port=3
  X : Outport  Port=4
  wires:
  g/1 -> MATLAB Function/4(g)
  u/1 -> Sum/2
  dq0/1 -> Integrator/2
  Integrator1/1 -> q/1, MATLAB Function1/1(q), MATLAB Function3/1(q), MATLAB Function/2(q), MATLAB Function4/1(q), MATLAB Function5/1(q), MATLAB Function2/1(q)
  uA/1 -> MATLAB Function2/2(uA)
  MATLAB Function1/1(X) -> X/1
  Integrator/1 -> dq/1, MATLAB Function3/2(dq), MATLAB Function/1(dq)
  MATLAB Function3/1(dX) -> dX/1
  MATLAB Function2/1(u) -> Sum/1
  Sum/1 -> MATLAB Function/3(u)
  MATLAB Function/1(ddq_) -> Sum1/2
  q0/1 -> Integrator1/2
  Sum1/1 -> Integrator/1
  MATLAB Function/2(dq_) -> Sum2/2
  Sum2/1 -> Integrator1/1
  inject_ddX/1 -> MATLAB Function4/2(inject_ddX)
  inject_dX/1 -> MATLAB Function5/2(inject_dX)
  MATLAB Function4/1(inject_ddq) -> Sum1/1
  MATLAB Function5/1(inject_dq) -> Sum2/1

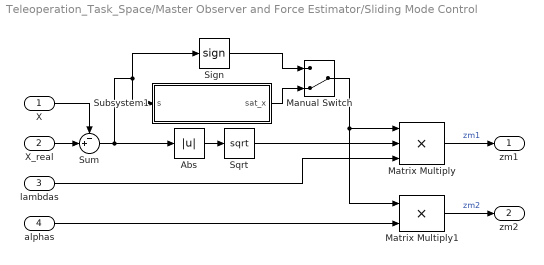
== system Teleoperation_Task_Space/Master Observer and Force Estimator/Sliding Mode Control ==
  X : Inport
  X_real : Inport  Port=2
  lambdas : Inport  Port=3
  alphas : Inport  Port=4
  Abs : Abs
  Manual Switch : ManualSwitch  CurrentSetting=0
  Matrix Multiply : Product  Inputs=***
  Matrix Multiply1 : Product
  Sign : Signum
  Sqrt : Sqrt  SaturateOnIntegerOverflow=on
  Subsystem1 : Subsystem
  Sum : Sum  Inputs=-+|
  zm1 : Outport
  zm2 : Outport  Port=2
  wires:
  Abs/1 -> Sqrt/1
  X/1 -> Sum/1
  lambdas/1 -> Matrix Multiply/3
  Sqrt/1 -> Matrix Multiply/2
  X_real/1 -> Sum/2
  Matrix Multiply/1 -> zm1/1  "zm1"
  Matrix Multiply1/1 -> zm2/1  "zm2"
  alphas/1 -> Matrix Multiply1/2
  Manual Switch/1 -> Matrix Multiply/1, Matrix Multiply1/1
  Sign/1 -> Manual Switch/1
  Subsystem1/1(sat_x) -> Manual Switch/2
  Sum/1 -> Sign/1, Subsystem1/1(s), Abs/1

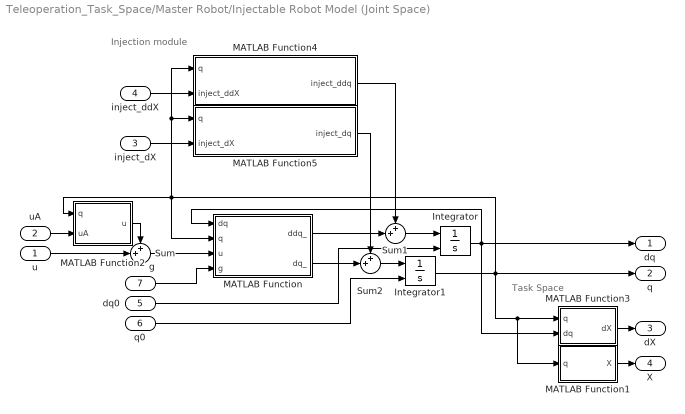
== system Teleoperation_Task_Space/Master Robot/Injectable Robot Model (Joint Space) ==
  note: Injection module
  note: Task Space
  u : Inport
  uA : Inport  Port=2
  inject_dX : Inport  Port=3
  inject_ddX : Inport  Port=4
  dq0 : Inport  Port=5
  q0 : Inport  Port=6
  g : Inport  Port=7
  Integrator : Integrator  InitialConditionSource=external  InitialCondition=x0
  Integrator1 : Integrator  InitialConditionSource=external  InitialCondition=x0
  MATLAB Function : MATLAB Function  TreatAsAtomicUnit=on
  MATLAB Function1 : MATLAB Function  TreatAsAtomicUnit=on
  MATLAB Function2 : MATLAB Function  TreatAsAtomicUnit=on
  MATLAB Function3 : MATLAB Function  TreatAsAtomicUnit=on
  MATLAB Function4 : MATLAB Function  TreatAsAtomicUnit=on
  MATLAB Function5 : MATLAB Function  TreatAsAtomicUnit=on
  Sum : Sum  Inputs=++|
  Sum1 : Sum  Inputs=++|
  Sum2 : Sum  Inputs=++|
  dq : Outport
  q : Outport  Port=2
  dX : Outport  Port=3
  X : Outport  Port=4
  wires:
  g/1 -> MATLAB Function/4(g)
  u/1 -> Sum/2
  dq0/1 -> Integrator/2
  Integrator1/1 -> q/1, MATLAB Function1/1(q), MATLAB Function3/1(q), MATLAB Function/2(q), MATLAB Function4/1(q), MATLAB Function5/1(q), MATLAB Function2/1(q)
  uA/1 -> MATLAB Function2/2(uA)
  MATLAB Function1/1(X) -> X/1
  Integrator/1 -> dq/1, MATLAB Function3/2(dq), MATLAB Function/1(dq)
  MATLAB Function3/1(dX) -> dX/1
  MATLAB Function2/1(u) -> Sum/1
  Sum/1 -> MATLAB Function/3(u)
  MATLAB Function/1(ddq_) -> Sum1/2
  q0/1 -> Integrator1/2
  Sum1/1 -> Integrator/1
  MATLAB Function/2(dq_) -> Sum2/2
  Sum2/1 -> Integrator1/1
  inject_ddX/1 -> MATLAB Function4/2(inject_ddX)
  inject_dX/1 -> MATLAB Function5/2(inject_dX)
  MATLAB Function4/1(inject_ddq) -> Sum1/1
  MATLAB Function5/1(inject_dq) -> Sum2/1

== system Teleoperation_Task_Space/Sensors/Compare Sensors ==
  Xm : Inport
  dXm : Inport  Port=2
  Xd : Inport  Port=3
  Xs : Inport  Port=4
  dXs : Inport  Port=5
  Bus Selector : BusSelector  OutputSignals=Xd,dXd
  Speed : Subsystem
      settings: PortSchema="{\"entries\":[{\"content\":{\"sides\":[{\"content\":{\"connectorIds\":[\"In1\",\"In2\"]},\"type\":\"ConnectorPlacement.EquallySpacedRectSide\",\"uuid\":\"98f8c5d8-e26e-427c-a81e-60bbe3a3ab4d\"},{\"content\":{\"connectorIds\":[\"In3\"],\"side\":\"RIGHT\"},\"type\":\"ConnectorPlacement.EquallySpacedRectSide\",\"uuid\":\"a51aa647-09cd-4fb3-b31a-f2bc2bc6e0ff\"},{\"content\":{\"connectorIds\":[],\"side\":\"TOP\"},\"type\":\"ConnectorPlacement.EquallySpacedRectSide\",\"uuid\":\"9387bbe5-2fda-43cb-b346-55f243092f42\"}]},\"type\":\"ConnectorPlacement.EquallySpacedConnector\",\"uuid\":\"8debe184-3b59-4f16-84f4-2d6030e17ba5\"}],\"packageUris\":[\"http://schema.mathworks.com/mf0/Connector/R2020b\"],\"version\":\"1.0\"}"
  State : Subsystem
      settings: PortSchema="{\"entries\":[{\"content\":{\"sides\":[{\"content\":{\"connectorIds\":[\"In1\",\"In2\"]},\"type\":\"ConnectorPlacement.EquallySpacedRectSide\",\"uuid\":\"01454c74-c00d-4dd4-8c17-6c92618f4fbd\"},{\"content\":{\"connectorIds\":[\"In3\"],\"side\":\"RIGHT\"},\"type\":\"ConnectorPlacement.EquallySpacedRectSide\",\"uuid\":\"513d8441-bd24-4ed7-81a7-c82fc02bd3bb\"},{\"content\":{\"connectorIds\":[],\"side\":\"TOP\"},\"type\":\"ConnectorPlacement.EquallySpacedRectSide\",\"uuid\":\"4be79af5-4243-4163-abc5-606cf31df7a9\"}]},\"type\":\"ConnectorPlacement.EquallySpacedConnector\",\"uuid\":\"51183099-fb0d-4d24-85ba-eaa305fd4a40\"}],\"packageUris\":[\"http://schema.mathworks.com/mf0/Connector/R2020b\"],\"version\":\"1.0\"}"
  wires:
  dXm/1 -> Speed/2(dm_in)
  dXs/1 -> Speed/3(ds_in)
  Xm/1 -> State/1(Xm^_in)
  Xs/1 -> State/3(Xs^_in)
  Xd/1 -> Bus Selector/1
  Bus Selector/1 -> State/2(Xd_in)  "<Xd>"
  Bus Selector/2 -> Speed/1(dd_in)  "<dXd>"

== system Teleoperation_Task_Space/Sensors/Master Desired Pose ==
  Bus Creator : BusCreator  Inputs=2
  Constant1 : Constant  Value=zeros(1,dh.dof_task)
  Constant2 : Constant  Value=zeros(1,dh.dof_task)
  Xd : Outport
  wires:
  Constant2/1 -> Bus Creator/2  "dXd"
  Constant1/1 -> Bus Creator/1  "Xd"
  Bus Creator/1 -> Xd/1

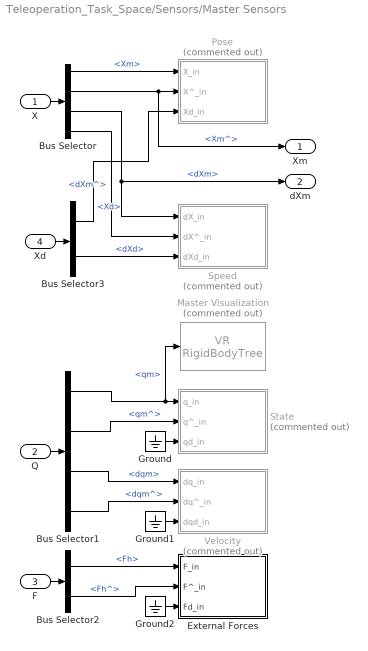
== system Teleoperation_Task_Space/Sensors/Master Sensors ==
  X : Inport
  Q : Inport  Port=2
  F : Inport  Port=3
  Xd : Inport  Port=4
  Bus Selector : BusSelector  OutputSignals=Xm,Xm^,dXm,dXm^
  Bus Selector1 : BusSelector  OutputSignals=qm,qm^,dqm,dqm^
  Bus Selector2 : BusSelector  OutputSignals=Fh,Fh^
  Bus Selector3 : BusSelector  OutputSignals=Xd,dXd
  External Forces : Subsystem
  Ground : Ground
  Ground1 : Ground
  Ground2 : Ground
  Master Visualization : vrlib/VR RigidBodyTree  Commented=on  RBT=UR5_robot  useRBT=on  Ts=-1  ForceViewerOpen=on
      settings: SourceProductBaseCode=SL
  Pose : Subsystem  Commented=on
  Speed : Subsystem  Commented=on
  State : Subsystem  Commented=on
  Velocity : Subsystem  Commented=on
  Xm : Outport
  dXm : Outport  Port=2
  wires:
  Bus Selector1/2 -> State/2(q^_in)  "<qm^>"
  Bus Selector1/3 -> Velocity/1(dq_in)  "<dqm>"
  Bus Selector2/2 -> External Forces/2(F^_in)  "<Fh^>"
  Bus Selector1/4 -> Velocity/2(dq^_in)  "<dqm^>"
  Ground/1 -> State/3(qd_in)
  Ground1/1 -> Velocity/3(dqd_in)
  Bus Selector/1 -> Pose/1(X_in)  "<Xm>"
  Bus Selector/3 -> dXm/1, Speed/1(dX_in)  "<dXm>"
  Bus Selector/4 -> Speed/2(dX^_in)  "<dXm^>"
  X/1 -> Bus Selector/1
  Bus Selector/2 -> Xm/1, Pose/2(X^_in)  "<Xm^>"
  Q/1 -> Bus Selector1/1
  Bus Selector1/1 -> Master Visualization/1, State/1(q_in)  "<qm>"
  F/1 -> Bus Selector2/1
  Bus Selector2/1 -> External Forces/1(F_in)  "<Fh>"
  Ground2/1 -> External Forces/3(Fd_in)
  Bus Selector3/1 -> Pose/3(Xd_in)  "<Xd>"
  Bus Selector3/2 -> Speed/3(dXd_in)  "<dXd>"
  Xd/1 -> Bus Selector3/1

== system Teleoperation_Task_Space/Sensors/Slave Desired Pose ==
  Bus Creator : BusCreator  Inputs=2
  Constant1 : Constant  Value=zeros(1,dh.dof_task)
  Constant2 : Constant  Value=zeros(1,dh.dof_task)
  Xd : Outport
  wires:
  Constant2/1 -> Bus Creator/2  "dXd"
  Constant1/1 -> Bus Creator/1  "Xd"
  Bus Creator/1 -> Xd/1

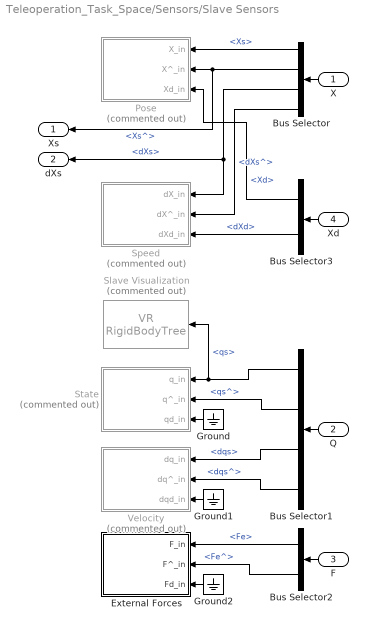
== system Teleoperation_Task_Space/Sensors/Slave Sensors ==
  X : Inport
  Q : Inport  Port=2
  F : Inport  Port=3
  Xd : Inport  Port=4
  Bus Selector : BusSelector  OutputSignals=Xs,Xs^,dXs,dXs^
  Bus Selector1 : BusSelector  OutputSignals=qs,qs^,dqs,dqs^
  Bus Selector2 : BusSelector  OutputSignals=Fe,Fe^
  Bus Selector3 : BusSelector  OutputSignals=Xd,dXd
  External Forces : Subsystem
  Ground : Ground
  Ground1 : Ground
  Ground2 : Ground
  Pose : Subsystem  Commented=on
  Slave Visualization : vrlib/VR RigidBodyTree  Commented=on  RBT=UR5_robot  useRBT=on  Ts=-1  ForceViewerOpen=on
      settings: SourceProductBaseCode=SL
  Speed : Subsystem  Commented=on
  State : Subsystem  Commented=on
  Velocity : Subsystem  Commented=on
  Xs : Outport
  dXs : Outport  Port=2
  wires:
  Bus Selector1/2 -> State/2(q^_in)  "<qs^>"
  Bus Selector1/3 -> Velocity/1(dq_in)  "<dqs>"
  Bus Selector2/2 -> External Forces/2(F^_in)  "<Fe^>"
  Bus Selector1/4 -> Velocity/2(dq^_in)  "<dqs^>"
  Ground/1 -> State/3(qd_in)
  Ground1/1 -> Velocity/3(dqd_in)
  Bus Selector/1 -> Pose/1(X_in)  "<Xs>"
  Bus Selector/3 -> dXs/1, Speed/1(dX_in)  "<dXs>"
  Bus Selector/4 -> Speed/2(dX^_in)  "<dXs^>"
  Bus Selector3/1 -> Pose/3(Xd_in)  "<Xd>"
  Bus Selector3/2 -> Speed/3(dXd_in)  "<dXd>"
  X/1 -> Bus Selector/1
  Bus Selector/2 -> Xs/1, Pose/2(X^_in)  "<Xs^>"
  Q/1 -> Bus Selector1/1
  Bus Selector1/1 -> Slave Visualization/1, State/1(q_in)  "<qs>"
  F/1 -> Bus Selector2/1
  Bus Selector2/1 -> External Forces/1(F_in)  "<Fe>"
  Xd/1 -> Bus Selector3/1
  Ground2/1 -> External Forces/3(Fd_in)

== system Teleoperation_Task_Space/Slave Observer and Force Estimator/Filter ==
  In1 : Inport  Partition=on  PartitionDimension=1  PartitionWidth=1  PartitionOffset=0
  Filter : TransferFcn  Numerator=zdq_B  Denominator=zdq_A
  For Each : ForEach  DisableCoverage=on
  Out1 : Outport  ConcatenationDimension=1
  wires:
  In1/1 -> Filter/1
  Filter/1 -> Out1/1

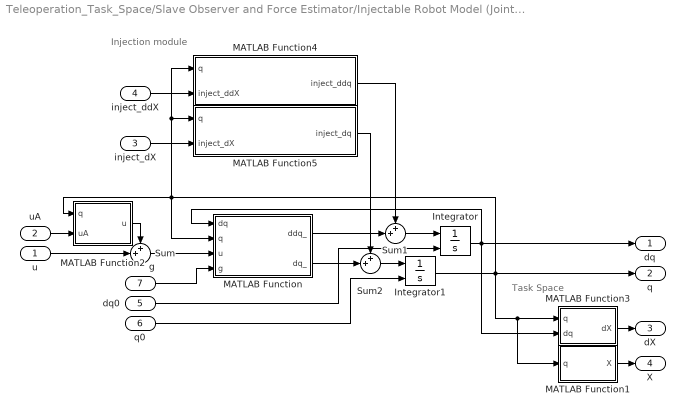
== system Teleoperation_Task_Space/Slave Observer and Force Estimator/Injectable Robot Model (Joint Space) ==
  note: Injection module
  note: Task Space
  u : Inport
  uA : Inport  Port=2
  inject_dX : Inport  Port=3
  inject_ddX : Inport  Port=4
  dq0 : Inport  Port=5
  q0 : Inport  Port=6
  g : Inport  Port=7
  Integrator : Integrator  InitialConditionSource=external  InitialCondition=x0
  Integrator1 : Integrator  InitialConditionSource=external  InitialCondition=x0
  MATLAB Function : MATLAB Function  TreatAsAtomicUnit=on
  MATLAB Function1 : MATLAB Function  TreatAsAtomicUnit=on
  MATLAB Function2 : MATLAB Function  TreatAsAtomicUnit=on
  MATLAB Function3 : MATLAB Function  TreatAsAtomicUnit=on
  MATLAB Function4 : MATLAB Function  TreatAsAtomicUnit=on
  MATLAB Function5 : MATLAB Function  TreatAsAtomicUnit=on
  Sum : Sum  Inputs=++|
  Sum1 : Sum  Inputs=++|
  Sum2 : Sum  Inputs=++|
  dq : Outport
  q : Outport  Port=2
  dX : Outport  Port=3
  X : Outport  Port=4
  wires:
  g/1 -> MATLAB Function/4(g)
  u/1 -> Sum/2
  dq0/1 -> Integrator/2
  Integrator1/1 -> q/1, MATLAB Function1/1(q), MATLAB Function3/1(q), MATLAB Function/2(q), MATLAB Function4/1(q), MATLAB Function5/1(q), MATLAB Function2/1(q)
  uA/1 -> MATLAB Function2/2(uA)
  MATLAB Function1/1(X) -> X/1
  Integrator/1 -> dq/1, MATLAB Function3/2(dq), MATLAB Function/1(dq)
  MATLAB Function3/1(dX) -> dX/1
  MATLAB Function2/1(u) -> Sum/1
  Sum/1 -> MATLAB Function/3(u)
  MATLAB Function/1(ddq_) -> Sum1/2
  q0/1 -> Integrator1/2
  Sum1/1 -> Integrator/1
  MATLAB Function/2(dq_) -> Sum2/2
  Sum2/1 -> Integrator1/1
  inject_ddX/1 -> MATLAB Function4/2(inject_ddX)
  inject_dX/1 -> MATLAB Function5/2(inject_dX)
  MATLAB Function4/1(inject_ddq) -> Sum1/1
  MATLAB Function5/1(inject_dq) -> Sum2/1

== system Teleoperation_Task_Space/Slave Observer and Force Estimator/Sliding Mode Control ==
  X : Inport
  X_real : Inport  Port=2
  lambdas : Inport  Port=3
  alphas : Inport  Port=4
  Abs : Abs
  Manual Switch : ManualSwitch  CurrentSetting=0
  Matrix Multiply : Product  Inputs=***
  Matrix Multiply1 : Product
  Sign : Signum
  Sqrt : Sqrt  SaturateOnIntegerOverflow=on
  Subsystem1 : Subsystem
  Sum : Sum  Inputs=-+|
  zm1 : Outport
  zm2 : Outport  Port=2
  wires:
  Abs/1 -> Sqrt/1
  X/1 -> Sum/1
  lambdas/1 -> Matrix Multiply/3
  Sqrt/1 -> Matrix Multiply/2
  X_real/1 -> Sum/2
  Matrix Multiply/1 -> zm1/1  "zm1"
  Matrix Multiply1/1 -> zm2/1  "zm2"
  alphas/1 -> Matrix Multiply1/2
  Manual Switch/1 -> Matrix Multiply/1, Matrix Multiply1/1
  Sign/1 -> Manual Switch/1
  Subsystem1/1(sat_x) -> Manual Switch/2
  Sum/1 -> Subsystem1/1(s), Sign/1, Abs/1

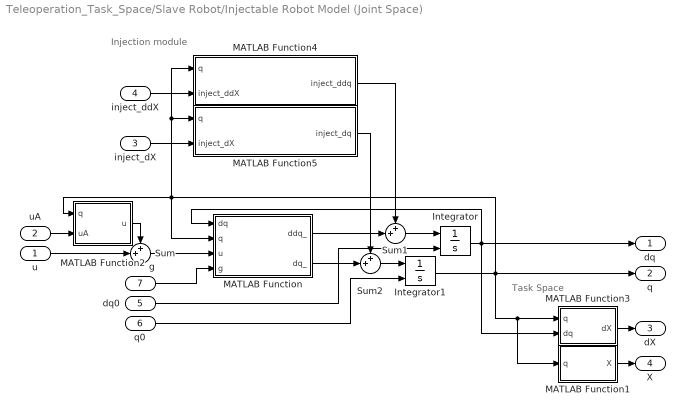
== system Teleoperation_Task_Space/Slave Robot/Injectable Robot Model (Joint Space) ==
  note: Injection module
  note: Task Space
  u : Inport
  uA : Inport  Port=2
  inject_dX : Inport  Port=3
  inject_ddX : Inport  Port=4
  dq0 : Inport  Port=5
  q0 : Inport  Port=6
  g : Inport  Port=7
  Integrator : Integrator  InitialConditionSource=external  InitialCondition=x0
  Integrator1 : Integrator  InitialConditionSource=external  InitialCondition=x0
  MATLAB Function : MATLAB Function  TreatAsAtomicUnit=on
  MATLAB Function1 : MATLAB Function  TreatAsAtomicUnit=on
  MATLAB Function2 : MATLAB Function  TreatAsAtomicUnit=on
  MATLAB Function3 : MATLAB Function  TreatAsAtomicUnit=on
  MATLAB Function4 : MATLAB Function  TreatAsAtomicUnit=on
  MATLAB Function5 : MATLAB Function  TreatAsAtomicUnit=on
  Sum : Sum  Inputs=++|
  Sum1 : Sum  Inputs=++|
  Sum2 : Sum  Inputs=++|
  dq : Outport
  q : Outport  Port=2
  dX : Outport  Port=3
  X : Outport  Port=4
  wires:
  g/1 -> MATLAB Function/4(g)
  u/1 -> Sum/2
  dq0/1 -> Integrator/2
  Integrator1/1 -> q/1, MATLAB Function1/1(q), MATLAB Function3/1(q), MATLAB Function/2(q), MATLAB Function4/1(q), MATLAB Function5/1(q), MATLAB Function2/1(q)
  uA/1 -> MATLAB Function2/2(uA)
  MATLAB Function1/1(X) -> X/1
  Integrator/1 -> dq/1, MATLAB Function3/2(dq), MATLAB Function/1(dq)
  MATLAB Function3/1(dX) -> dX/1
  MATLAB Function2/1(u) -> Sum/1
  Sum/1 -> MATLAB Function/3(u)
  MATLAB Function/1(ddq_) -> Sum1/2
  q0/1 -> Integrator1/2
  Sum1/1 -> Integrator/1
  MATLAB Function/2(dq_) -> Sum2/2
  Sum2/1 -> Integrator1/1
  inject_ddX/1 -> MATLAB Function4/2(inject_ddX)
  inject_dX/1 -> MATLAB Function5/2(inject_dX)
  MATLAB Function4/1(inject_ddq) -> Sum1/1
  MATLAB Function5/1(inject_dq) -> Sum2/1

== system Teleoperation_Task_Space/Slave controller/Slave Command Filter ==
  In1 : Inport  Partition=on  PartitionDimension=1  PartitionWidth=1  PartitionOffset=0
  Filter : TransferFcn  Numerator=Fs_B  Denominator=Fs_A
  For Each : ForEach  DisableCoverage=on
  Out1 : Outport  ConcatenationDimension=1
  wires:
  In1/1 -> Filter/1
  Filter/1 -> Out1/1

== system Teleoperation_Task_Space/Slave controller/Sliding Surface ==
  e : Inport
  de : Inport  Port=2
  f : Inport  Port=3
  Integrator : Integrator
  Multiply1 : Gain  Gain=B_s  Multiplication=Matrix(K*u)
  Multiply2 : Gain  Gain=K_s  Multiplication=Matrix(K*u)
  Multiply3 : Gain  Gain=inv(M_s)  Multiplication=Matrix(K*u)
  Sum : Sum  Inputs=|++
  Sum2 : Sum  Inputs=+++
  s : Outport
  wires:
  Multiply3/1 -> Integrator/1
  Integrator/1 -> Sum/1
  Sum2/1 -> Multiply3/1
  f/1 -> Sum2/1
  e/1 -> Multiply2/1
  Multiply2/1 -> Sum2/2
  de/1 -> Sum/2, Multiply1/1
  Multiply1/1 -> Sum2/3
  Sum/1 -> s/1

== system Teleoperation_Task_Space/Slave controller/Subsystem1 ==
  s : Inport
  Abs : Abs
  Constant : Constant  Value=10e-2
  Constant1 : Constant  Value=ones(1,dh.dof_task)
  Constant2 : Constant
  Divide : Product  Inputs=*/
  Product : Product
  Product1 : Product
  Relational Operator : RelationalOperator  Operator=>  OutDataTypeStr=boolean  RndMeth=Simplest
  Sign : Signum
  Sum : Sum  Inputs=+-|
  Sum1 : Sum  Inputs=+|+
  sat_x : Outport
  wires:
  Divide/1 -> Product1/2, Sign/1, Abs/1
  s/1 -> Divide/1
  Constant/1 -> Divide/2
  Abs/1 -> Relational Operator/1
  Sum1/1 -> sat_x/1
  Sign/1 -> Product/1
  Constant1/1 -> Relational Operator/2
  Relational Operator/1 -> Sum/2, Product/2
  Constant2/1 -> Sum/1
  Sum/1 -> Product1/1
  Product/1 -> Sum1/1
  Product1/1 -> Sum1/2

== system Teleoperation_Task_Space/Human (Task Space)/Motion Tracking control/Slave Position Filter ==
  In1 : Inport  Partition=on  PartitionDimension=1  PartitionWidth=1  PartitionOffset=0
  Filter : TransferFcn  Numerator=Fh_B  Denominator=Fh_A
  For Each : ForEach  DisableCoverage=on
  Out1 : Outport  ConcatenationDimension=1
  wires:
  In1/1 -> Filter/1
  Filter/1 -> Out1/1

== system Teleoperation_Task_Space/Human (Task Space)/Motion Tracking control/Slave Speed Filter ==
  In1 : Inport  Partition=on  PartitionDimension=1  PartitionWidth=1  PartitionOffset=0
  Filter : TransferFcn  Numerator=Fh_B  Denominator=Fh_A
  For Each : ForEach  DisableCoverage=on
  Out1 : Outport  ConcatenationDimension=1
  wires:
  In1/1 -> Filter/1
  Filter/1 -> Out1/1

== system Teleoperation_Task_Space/Master Observer and Force Estimator/Sliding Mode Control/Subsystem1 ==
  s : Inport
  Abs : Abs
  Constant : Constant  Value=10e-5
  Constant1 : Constant  Value=ones(1,dh.dof_task)
  Constant2 : Constant
  Divide : Product  Inputs=*/
  Product : Product
  Product1 : Product
  Relational Operator : RelationalOperator  Operator=>  OutDataTypeStr=boolean  RndMeth=Simplest
  Sign : Signum
  Sum : Sum  Inputs=+-|
  Sum1 : Sum  Inputs=+|+
  sat_x : Outport
  wires:
  Divide/1 -> Product1/2, Sign/1, Abs/1
  s/1 -> Divide/1
  Constant/1 -> Divide/2
  Abs/1 -> Relational Operator/1
  Sum1/1 -> sat_x/1
  Sign/1 -> Product/1
  Constant1/1 -> Relational Operator/2
  Relational Operator/1 -> Sum/2, Product/2
  Constant2/1 -> Sum/1
  Sum/1 -> Product1/1
  Product/1 -> Sum1/1
  Product1/1 -> Sum1/2

== system Teleoperation_Task_Space/Sensors/Compare Sensors/Speed ==
  dd_in : Inport
  dm_in : Inport  Port=2
  ds_in : Inport  Port=3
  Compare Speed : Scope  NumInputPorts=6
  Mux{,1..5} (6 alike) : Mux  Inputs=3
  dXd : Demux  Outputs=dh.dof
  dXm^ : Demux  Outputs=dh.dof
  dXs^ : Demux  Outputs=dh.dof
  wires:
  ds_in/1 -> dXs^/1
  dm_in/1 -> dXm^/1
  dd_in/1 -> dXd/1
  dXm^/5 -> Mux4/1
  dXs^/6 -> Mux5/3
  dXs^/5 -> Mux4/3
  dXs^/4 -> Mux3/3
  dXs^/2 -> Mux1/3
  dXd/6 -> Mux5/2
  dXd/3 -> Mux2/2
  dXd/5 -> Mux4/2
  dXd/4 -> Mux3/2
  dXs^/3 -> Mux2/3
  Mux3/1 -> Compare Speed/4
  Mux1/1 -> Compare Speed/2
  dXm^/6 -> Mux5/1
  dXm^/4 -> Mux3/1
  dXd/2 -> Mux1/2
  Mux5/1 -> Compare Speed/6
  Mux2/1 -> Compare Speed/3
  dXd/1 -> Mux/2
  dXs^/1 -> Mux/3
  Mux/1 -> Compare Speed/1
  dXm^/3 -> Mux2/1
  Mux4/1 -> Compare Speed/5
  dXm^/1 -> Mux/1
  dXm^/2 -> Mux1/1

== system Teleoperation_Task_Space/Sensors/Compare Sensors/State ==
  Xm^_in : Inport
  Xd_in : Inport  Port=2
  Xs^_in : Inport  Port=3
  Compare State : Scope  NumInputPorts=6
  Mux{,1..5} (6 alike) : Mux  Inputs=3
  Xd : Demux  Outputs=dh.dof
  Xm^ : Demux  Outputs=dh.dof
  Xs^ : Demux  Outputs=dh.dof
  wires:
  Mux5/1 -> Compare State/6
  Xm^/2 -> Mux1/1
  Xm^/3 -> Mux2/1
  Xs^/3 -> Mux2/3
  Xd/1 -> Mux/2
  Xs^/4 -> Mux3/3
  Xm^/1 -> Mux/1
  Mux4/1 -> Compare State/5
  Xs^/5 -> Mux4/3
  Mux/1 -> Compare State/1
  Xd/4 -> Mux3/2
  Xs^/1 -> Mux/3
  Xs^/2 -> Mux1/3
  Mux2/1 -> Compare State/3
  Xd/6 -> Mux5/2
  Xm^/5 -> Mux4/1
  Xs^/6 -> Mux5/3
  Xd/2 -> Mux1/2
  Mux1/1 -> Compare State/2
  Xm^/4 -> Mux3/1
  Mux3/1 -> Compare State/4
  Xm^/6 -> Mux5/1
  Xd/5 -> Mux4/2
  Xd/3 -> Mux2/2
  Xs^_in/1 -> Xs^/1
  Xd_in/1 -> Xd/1
  Xm^_in/1 -> Xm^/1
